simulink model "TP2sim"  (R2020b)
settings: Solver=VariableStepAuto  StartTime=0.0  StopTime=15  MaxStep=0.1  RelTol=1e-3
values from neighbouring files (symbols this model uses):
  K = 5    [TP2m.m]
  Kinconnu = DeltaY/DeltaU    (= 2.3)    [TP2m.m]
  kp = 5/K    (= 1)    [TP2m.m]
  out1 = flip(out1)    [TD2m.m]
  out2 = flip(out2)    [TD2m.m]
  tau = 3    [TP2m.m]
  tauinconnu = t1-t0    (= 1.252)    [TP2m.m]
  Td = 0    [TP2m.m]
  Te = 0.5    [TD2m.m]    (also in TP2m.m = 0.6)
  Ti = tau    (= 3)    [TP2m.m]
libraries: pid_lib x3
settings Model: Creator=Etudiants  LastModifiedBy=Etudiants

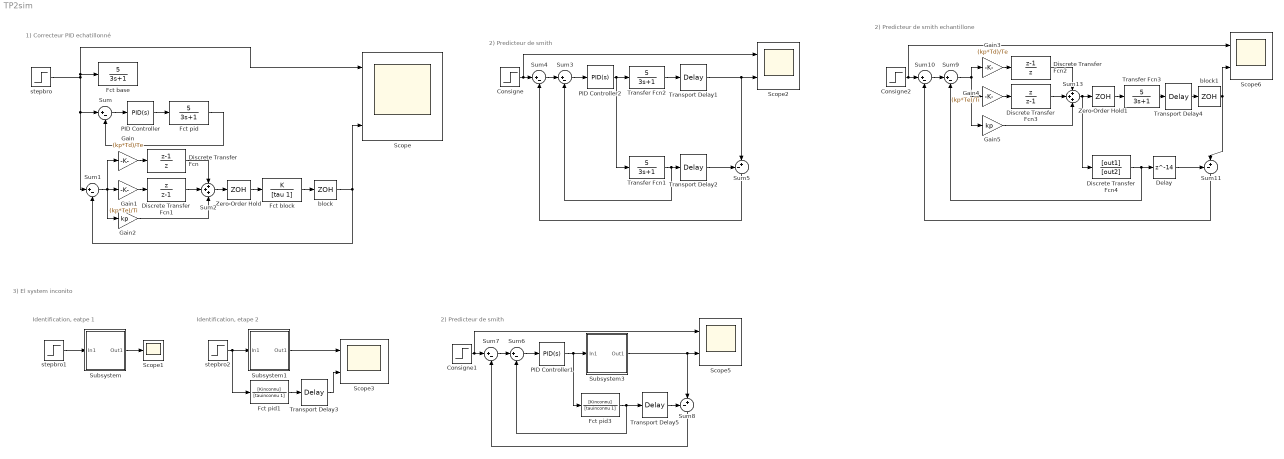
== system TP2sim ==
  note: Identification, eatpe 1
  note: 1) Correcteur PID echatillonné
  note: 2) Predicteur de smith
  note: 3) El system inconito
  note: Identification, etape 2
  note: 2) Predicteur de smith
  note: 2) Predicteur de smith echantillone
  Consigne : Step  SampleTime=0
  Consigne1 : Step  SampleTime=0
  Consigne2 : Step  SampleTime=0
  Delay : Delay  DelayLength=14
  Discrete Transfer Fcn : DiscreteTransferFcn  Numerator=[1 -1]  Denominator=[1 0]  SampleTime=3/5
  Discrete Transfer Fcn1 : DiscreteTransferFcn  Numerator=[1 0]  Denominator=[1 -1]  SampleTime=3/5
  Discrete Transfer Fcn2 : DiscreteTransferFcn  Numerator=[1 -1]  Denominator=[1 0]  SampleTime=3/5
  Discrete Transfer Fcn3 : DiscreteTransferFcn  Numerator=[1 0]  Denominator=[1 -1]  SampleTime=3/5
  Discrete Transfer Fcn4 : DiscreteTransferFcn  Numerator=[out1]  Denominator=[out2]  SampleTime=Te
  Fct base : TransferFcn  Numerator=[5]  Denominator=[3 1]
  Fct block : TransferFcn  Numerator=K  Denominator=[tau 1]
  Fct pid : TransferFcn  Numerator=[5]  Denominator=[3 1]
  Fct pid1 : TransferFcn  Numerator=[Kinconnu]  Denominator=[tauinconnu 1]
  Fct pid3 : TransferFcn  Numerator=[Kinconnu]  Denominator=[tauinconnu 1]
  Gain : Gain  Gain=(kp*Td)/Te
  Gain1 : Gain  Gain=(kp*Te)/Ti
  Gain2 : Gain  Gain=kp
  Gain3 : Gain  Gain=(kp*Td)/Te
  Gain4 : Gain  Gain=(kp*Te)/Ti
  Gain5 : Gain  Gain=kp
  PID Controller : pid_lib/PID Controller  Controller=PID  Form=Parallel  TimeDomain=Continuous-time  UseExternalTs=off  SampleTime=-1  IntegratorMethod=Forward Euler  FilterMethod=Forward Euler  ControllerParametersSource=internal  P=1  I=1/3  D=0  UseFilter=on  N=100  TunerSelectOption=Transfer Function Based (PID Tuner App)  InitialConditionSource=internal  InitialConditionForIntegrator=0  InitialConditionForFilter=0  DifferentiatorICPrevScaledInput=0  ExternalReset=none  TrackingMode=off  Kt=1  LimitOutput=off  SatLimitsSource=internal  UpperSaturationLimit=inf  LowerSaturationLimit=-inf  LinearizeAsGain=on  AntiWindupMode=none  Kb=1  POutMin=[]  POutMax=[]  IOutMin=[]  IOutMax=[]  DOutMin=[]  DOutMax=[]  NOutMin=[]  NOutMax=[]  SumOutMin=[]  SumOutMax=[]  SaturationOutMin=[]  SaturationOutMax=[]  PParamMin=[]  PParamMax=[]  IParamMin=[]  IParamMax=[]  DParamMin=[]  DParamMax=[]  NParamMin=[]  NParamMax=[]  KbParamMin=[]  KbParamMax=[]  KtParamMin=[]  KtParamMax=[]  KbOutMin=[]  KbOutMax=[]  KtOutMin=[]  KtOutMax=[]  IntegratorOutMin=[]  IntegratorOutMax=[]  FilterOutMin=[]  FilterOutMax=[]  SumI1OutMin=[]  SumI1OutMax=[]  SumI2OutMin=[]  SumI2OutMax=[]  SumI3OutMin=[]  SumI3OutMax=[]  SumI4OutMin=[]  SumI4OutMax=[]  SumDOutMin=[]  SumDOutMax=[]  DifferentiatorOutMin=[]  DifferentiatorOutMax=[]  FilterDiffOutCoefMin=[]  FilterDiffOutCoefMax=[]  ReciprocalOutMin=[]  ReciprocalOutMax=[]  SumDenOutMin=[]  SumDenOutMax=[]  SumNumOutMin=[]  SumNumOutMax=[]  DivideOutMin=[]  DivideOutMax=[]  UdiffTsProdOutMin=[]  UdiffTsProdOutMax=[]  NTsProdOutMin=[]  NTsProdOutMax=[]  UintegralTsProdOutMin=[]  UintegralTsProdOutMax=[]  UngainTsProdOutMin=[]  UngainTsProdOutMax=[]  IntegratorContinuousStateAttributes=''  IntegratorStateMustResolveToSignalObject=off  IntegratorRTWStateStorageClass=Auto  FilterContinuousStateAttributes=''  FilterStateMustResolveToSignalObject=off  FilterRTWStateStorageClass=Auto  ParallelPVariant=InternalParameters  IdealPVariant=Disabled  IVariant=InternalParameters  DVariant=InternalParameters  IntegratorVariant=Continuous  SatVariant=Disabled  AWVariant=Passthrough  PCopyVariant=Disabled  TRVariant=Disabled  FdbkBlocksVariant=Forward  IdealPFdbkVariant=Disabled  SatFdbkVariant=Disabled  DerivativeFilterVariant=ContFilter  NVariant=InternalParameters  NCopyVariant=Disabled  FilterICVariant=InternalICsFilter  IntegratorICVariant=InternalICs  ExternalResetVariant=Disabled  TRSumVariant=Passthrough  SumFdbkVariant=Disabled  SumVariant=Sum_PID  TsampFilterVariant=InternalTs  TsampNgainVariant=Passthrough  TsampIntegralVariant=Passthrough  ExternalSaturationOutDataTypeStr=Inherit: Same as second input
  PID Controller1 : pid_lib/PID Controller  Controller=PID  Form=Ideal  TimeDomain=Continuous-time  UseExternalTs=off  SampleTime=-1  IntegratorMethod=Forward Euler  FilterMethod=Forward Euler  ControllerParametersSource=internal  P=5/Kinconnu  I=1/tauinconnu  D=0  UseFilter=on  N=100  TunerSelectOption=Transfer Function Based (PID Tuner App)  InitialConditionSource=internal  InitialConditionForIntegrator=0  InitialConditionForFilter=0  DifferentiatorICPrevScaledInput=0  ExternalReset=none  TrackingMode=off  Kt=1  LimitOutput=off  SatLimitsSource=internal  UpperSaturationLimit=inf  LowerSaturationLimit=-inf  LinearizeAsGain=on  AntiWindupMode=none  Kb=1  POutMin=[]  POutMax=[]  IOutMin=[]  IOutMax=[]  DOutMin=[]  DOutMax=[]  NOutMin=[]  NOutMax=[]  SumOutMin=[]  SumOutMax=[]  SaturationOutMin=[]  SaturationOutMax=[]  PParamMin=[]  PParamMax=[]  IParamMin=[]  IParamMax=[]  DParamMin=[]  DParamMax=[]  NParamMin=[]  NParamMax=[]  KbParamMin=[]  KbParamMax=[]  KtParamMin=[]  KtParamMax=[]  KbOutMin=[]  KbOutMax=[]  KtOutMin=[]  KtOutMax=[]  IntegratorOutMin=[]  IntegratorOutMax=[]  FilterOutMin=[]  FilterOutMax=[]  SumI1OutMin=[]  SumI1OutMax=[]  SumI2OutMin=[]  SumI2OutMax=[]  SumI3OutMin=[]  SumI3OutMax=[]  SumI4OutMin=[]  SumI4OutMax=[]  SumDOutMin=[]  SumDOutMax=[]  DifferentiatorOutMin=[]  DifferentiatorOutMax=[]  FilterDiffOutCoefMin=[]  FilterDiffOutCoefMax=[]  ReciprocalOutMin=[]  ReciprocalOutMax=[]  SumDenOutMin=[]  SumDenOutMax=[]  SumNumOutMin=[]  SumNumOutMax=[]  DivideOutMin=[]  DivideOutMax=[]  UdiffTsProdOutMin=[]  UdiffTsProdOutMax=[]  NTsProdOutMin=[]  NTsProdOutMax=[]  UintegralTsProdOutMin=[]  UintegralTsProdOutMax=[]  UngainTsProdOutMin=[]  UngainTsProdOutMax=[]  IntegratorContinuousStateAttributes=''  IntegratorStateMustResolveToSignalObject=off  IntegratorRTWStateStorageClass=Auto  FilterContinuousStateAttributes=''  FilterStateMustResolveToSignalObject=off  FilterRTWStateStorageClass=Auto  ParallelPVariant=Passthrough  IdealPVariant=InternalParameters  IVariant=InternalParameters  DVariant=InternalParameters  IntegratorVariant=Continuous  SatVariant=Disabled  AWVariant=Passthrough  PCopyVariant=Disabled  TRVariant=Disabled  FdbkBlocksVariant=Forward  IdealPFdbkVariant=Disabled  SatFdbkVariant=Disabled  DerivativeFilterVariant=ContFilter  NVariant=InternalParameters  NCopyVariant=Disabled  FilterICVariant=InternalICsFilter  IntegratorICVariant=InternalICs  ExternalResetVariant=Disabled  TRSumVariant=Passthrough  SumFdbkVariant=Disabled  SumVariant=Sum_PID  TsampFilterVariant=InternalTs  TsampNgainVariant=Passthrough  TsampIntegralVariant=Passthrough  ExternalSaturationOutDataTypeStr=Inherit: Same as second input
  PID Controller2 : pid_lib/PID Controller  Controller=PID  Form=Ideal  TimeDomain=Continuous-time  UseExternalTs=off  SampleTime=-1  IntegratorMethod=Forward Euler  FilterMethod=Forward Euler  ControllerParametersSource=internal  P=1  I=1/3  D=0  UseFilter=on  N=100  TunerSelectOption=Transfer Function Based (PID Tuner App)  InitialConditionSource=internal  InitialConditionForIntegrator=0  InitialConditionForFilter=0  DifferentiatorICPrevScaledInput=0  ExternalReset=none  TrackingMode=off  Kt=1  LimitOutput=off  SatLimitsSource=internal  UpperSaturationLimit=inf  LowerSaturationLimit=-inf  LinearizeAsGain=on  AntiWindupMode=none  Kb=1  POutMin=[]  POutMax=[]  IOutMin=[]  IOutMax=[]  DOutMin=[]  DOutMax=[]  NOutMin=[]  NOutMax=[]  SumOutMin=[]  SumOutMax=[]  SaturationOutMin=[]  SaturationOutMax=[]  PParamMin=[]  PParamMax=[]  IParamMin=[]  IParamMax=[]  DParamMin=[]  DParamMax=[]  NParamMin=[]  NParamMax=[]  KbParamMin=[]  KbParamMax=[]  KtParamMin=[]  KtParamMax=[]  KbOutMin=[]  KbOutMax=[]  KtOutMin=[]  KtOutMax=[]  IntegratorOutMin=[]  IntegratorOutMax=[]  FilterOutMin=[]  FilterOutMax=[]  SumI1OutMin=[]  SumI1OutMax=[]  SumI2OutMin=[]  SumI2OutMax=[]  SumI3OutMin=[]  SumI3OutMax=[]  SumI4OutMin=[]  SumI4OutMax=[]  SumDOutMin=[]  SumDOutMax=[]  DifferentiatorOutMin=[]  DifferentiatorOutMax=[]  FilterDiffOutCoefMin=[]  FilterDiffOutCoefMax=[]  ReciprocalOutMin=[]  ReciprocalOutMax=[]  SumDenOutMin=[]  SumDenOutMax=[]  SumNumOutMin=[]  SumNumOutMax=[]  DivideOutMin=[]  DivideOutMax=[]  UdiffTsProdOutMin=[]  UdiffTsProdOutMax=[]  NTsProdOutMin=[]  NTsProdOutMax=[]  UintegralTsProdOutMin=[]  UintegralTsProdOutMax=[]  UngainTsProdOutMin=[]  UngainTsProdOutMax=[]  IntegratorContinuousStateAttributes=''  IntegratorStateMustResolveToSignalObject=off  IntegratorRTWStateStorageClass=Auto  FilterContinuousStateAttributes=''  FilterStateMustResolveToSignalObject=off  FilterRTWStateStorageClass=Auto  ParallelPVariant=Passthrough  IdealPVariant=InternalParameters  IVariant=InternalParameters  DVariant=InternalParameters  IntegratorVariant=Continuous  SatVariant=Disabled  AWVariant=Passthrough  PCopyVariant=Disabled  TRVariant=Disabled  FdbkBlocksVariant=Forward  IdealPFdbkVariant=Disabled  SatFdbkVariant=Disabled  DerivativeFilterVariant=ContFilter  NVariant=InternalParameters  NCopyVariant=Disabled  FilterICVariant=InternalICsFilter  IntegratorICVariant=InternalICs  ExternalResetVariant=Disabled  TRSumVariant=Passthrough  SumFdbkVariant=Disabled  SumVariant=Sum_PID  TsampFilterVariant=InternalTs  TsampNgainVariant=Passthrough  TsampIntegralVariant=Passthrough  ExternalSaturationOutDataTypeStr=Inherit: Same as second input
  Scope : Scope  NumInputPorts=3
  Scope1 : Scope
  Scope{2..3,5..6} (4 alike) : Scope  NumInputPorts=2
  Subsystem : Subsystem
  Subsystem1 : Subsystem
  Subsystem3 : Subsystem
  Sum{,1,3..4,6..7,9..10} (8 alike) : Sum  Inputs=|+-
  Sum11 : Sum  Inputs=-+|
  Sum13 : Sum  Inputs=+++
  Sum2 : Sum  Inputs=+++
  Sum5 : Sum  Inputs=-+|
  Sum8 : Sum  Inputs=-+|
  Transfer Fcn1 : TransferFcn  Numerator=[5]  Denominator=[3 1]
  Transfer Fcn2 : TransferFcn  Numerator=[5]  Denominator=[3 1]
  Transfer Fcn3 : TransferFcn  Numerator=[5]  Denominator=[3 1]
  Transport Delay1 : TransportDelay  DelayTime=7
  Transport Delay2 : TransportDelay  DelayTime=7
  Transport Delay3 : TransportDelay  DelayTime=2.1
  Transport Delay4 : TransportDelay  DelayTime=7
  Transport Delay5 : TransportDelay  DelayTime=2.1
  Zero-Order Hold : ZeroOrderHold  SampleTime=Te
  Zero-Order Hold1 : ZeroOrderHold  SampleTime=Te
  block : ZeroOrderHold  SampleTime=Te
  block1 : ZeroOrderHold  SampleTime=Te
  stepbro : Step  SampleTime=0
  stepbro1 : Step  SampleTime=0
  stepbro2 : Step  SampleTime=0
  wires:
  PID Controller/1 -> Fct pid/1
  Fct pid/1 -> Sum/2
  Sum/1 -> PID Controller/1
  stepbro/1 -> Scope/1, Fct base/1, Sum1/1, Sum/1
  Sum1/1 -> Gain2/1, Gain/1, Gain1/1
  Fct block/1 -> block/1
  block/1 -> Scope/3, Sum1/2
  Sum2/1 -> Zero-Order Hold/1
  Zero-Order Hold/1 -> Fct block/1
  Gain/1 -> Discrete Transfer Fcn/1
  Gain1/1 -> Discrete Transfer Fcn1/1
  Discrete Transfer Fcn1/1 -> Sum2/2
  Discrete Transfer Fcn/1 -> Sum2/1
  Gain2/1 -> Sum2/3
  Transfer Fcn1/1 -> Sum3/2, Transport Delay2/1
  Sum4/1 -> Sum3/1
  Transport Delay2/1 -> Sum5/1
  Consigne/1 -> Scope2/1, Sum4/1
  PID Controller2/1 -> Transfer Fcn2/1, Transfer Fcn1/1
  Transport Delay1/1 -> Sum5/2, Scope2/2
  Sum3/1 -> PID Controller2/1
  Sum5/1 -> Sum4/2
  Transfer Fcn2/1 -> Transport Delay1/1
  stepbro1/1 -> Subsystem/1(In1)
  Subsystem/1(Out1) -> Scope1/1
  Subsystem1/1(Out1) -> Scope3/1
  stepbro2/1 -> Fct pid1/1, Subsystem1/1(In1)
  Transport Delay3/1 -> Scope3/2
  Fct pid1/1 -> Transport Delay3/1
  Sum8/1 -> Sum7/2
  Subsystem3/1(Out1) -> Scope5/2, Sum8/2
  Consigne1/1 -> Scope5/1, Sum7/1
  Fct pid3/1 -> Transport Delay5/1, Sum6/2
  Transport Delay5/1 -> Sum8/1
  PID Controller1/1 -> Subsystem3/1(In1), Fct pid3/1
  Sum6/1 -> PID Controller1/1
  Sum7/1 -> Sum6/1
  Sum11/1 -> Sum10/2
  Consigne2/1 -> Scope6/1, Sum10/1
  Discrete Transfer Fcn4/1 -> Delay/1, Sum9/2
  Delay/1 -> Sum11/1
  Sum10/1 -> Sum9/1
  Zero-Order Hold1/1 -> Transfer Fcn3/1
  Sum13/1 -> Discrete Transfer Fcn4/1, Zero-Order Hold1/1
  Gain5/1 -> Sum13/3
  Gain4/1 -> Discrete Transfer Fcn3/1
  Discrete Transfer Fcn3/1 -> Sum13/2
  Gain3/1 -> Discrete Transfer Fcn2/1
  Discrete Transfer Fcn2/1 -> Sum13/1
  Sum9/1 -> Gain5/1, Gain4/1, Gain3/1
  block1/1 -> Sum11/2, Scope6/2
  Transfer Fcn3/1 -> Transport Delay4/1
  Transport Delay4/1 -> block1/1

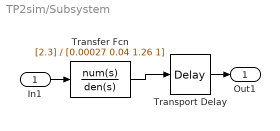
== system TP2sim/Subsystem ==
  In1 : Inport
  Transfer Fcn : TransferFcn  Numerator=[2.3]  Denominator=[0.00027 0.04 1.26 1]
  Transport Delay : TransportDelay  DelayTime=2.1  BufferSize=10024
  Out1 : Outport
  wires:
  In1/1 -> Transfer Fcn/1
  Transport Delay/1 -> Out1/1
  Transfer Fcn/1 -> Transport Delay/1

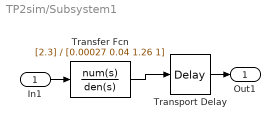
== system TP2sim/Subsystem1 ==
  In1 : Inport
  Transfer Fcn : TransferFcn  Numerator=[2.3]  Denominator=[0.00027 0.04 1.26 1]
  Transport Delay : TransportDelay  DelayTime=2.1  BufferSize=10024
  Out1 : Outport
  wires:
  In1/1 -> Transfer Fcn/1
  Transport Delay/1 -> Out1/1
  Transfer Fcn/1 -> Transport Delay/1

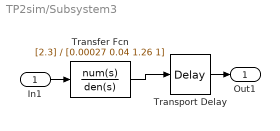
== system TP2sim/Subsystem3 ==
  In1 : Inport
  Transfer Fcn : TransferFcn  Numerator=[2.3]  Denominator=[0.00027 0.04 1.26 1]
  Transport Delay : TransportDelay  DelayTime=2.1  BufferSize=10024
  Out1 : Outport
  wires:
  In1/1 -> Transfer Fcn/1
  Transport Delay/1 -> Out1/1
  Transfer Fcn/1 -> Transport Delay/1
